simulink model "HEVPlant_Dummy"  (R2018b)
settings: configuration reference "Config_Plant" (kept outside this file)
PreLoadFcn:
  | HEVPlant_Ptbs_V1_BusInfo
model workspace (MAT data in the model file):
  DiffRatio = 3.421
  EV_current = 200
  EV_motion = [20 4 0.8]
  EV_sf = 2000
  EngDriveRatio = 0.813008130081
  Fs = 0
  Fv = 0.0025
  Jcomp = 0.0227
  Jengine = 0.22
  Ki = 251.3274
  Kisa = 346.6583
  Kp_d = 0.47149
  Kp_q = 0.52125
  Ksa = 85.4316
  Ksf = 1996.2651
  Ld = 0.0003752
  Ldq = [0.0003752 0.0004148]
  Lq = 0.0004148
  Mechanical = [0.0227 0.0025 0]
  MotGbRatio = 1
  P = 4
  PolePairs = 4
  RWheel = 0.3
  Rs = 0.2
  T_max = 120
  T_mtpa = [0 13.3131834767 26.6278836885 39.9456159322 53.2678926341 66.5962219318 79.9321062746 93.277041051 106.632513247 120.000000141]
  b_axle = Simulink.Parameter
  b_axle.Value = 10
  b_axle.DataType = 'auto'
  b_axle.Dimensions = [1 1]
  b_driveshaft = Simulink.Parameter
  b_driveshaft.Value = 10
  b_driveshaft.DataType = 'auto'
  b_driveshaft.Dimensions = [1 1]
  ba = 3.4029
  id_mtpa = [0 -0.114523352646 -0.457989076459 -1.03008464374 -1.83029075221 -2.85788367342 -4.11193850568 -5.59133329791 -7.29475400168 -9.22070020138]
  idq0 = [0 0]
  idq_limits = [-9.220699542 166.993501392 167.247872355]
  iq_mtpa = [0 18.5827440345 37.1633719111 55.7397734896 74.3098506185 92.871523015 111.422734008 129.961456105 148.485696337 166.993501356]
  k_axle = Simulink.Parameter
  k_axle.Value = 5000
  k_axle.DataType = 'auto'
  k_axle.Dimensions = [1 1]
  k_driveshaft = Simulink.Parameter
  k_driveshaft.Value = 1000
  k_driveshaft.DataType = 'auto'
  k_driveshaft.Dimensions = [1 1]
  lambda_pm = 0.1194
  mechanical = [0.0227 0.0025 0]
  mot.max_trq = 307
  mot.max_pwr = 124
  mot.spd = [0 500 1000 1500 2000 2500 3000 3500 3857.04487493 4000 4500 5000 5500 6000 6500 7000 7500 8000 8500 9000 9500 10000 10500 11000 11500 12000 12500]
  mot.trq = [307 307 307 307 307 307 307 307 307 296.028194151 263.136172579 236.822555321 215.29323211 197.352129434 182.171196401 169.158968086 157.881703547 148.014097075 139.307385483 131.568086289 124.643450169 118.41127766 112.772645391 107.646616055 102.9663284 98.676064717 94.7290221283]
  mot.trq_cp = [296.028194151 263.136172579 236.822555321 215.29323211 197.352129434 182.171196401 169.158968086 157.881703547 148.014097075 139.307385483 131.568086289 124.643450169 118.41127766 112.772645391 107.646616055 102.9663284 98.676064717 94.7290221283]
  mot.J = 0.02
  mot.damp = 0.0001
  mot.Tc = 0.0267
  mot.map.spdindex = [0 1000 2000 3000 3857 4000 5000 6000 7000 8000 9000 10000 11000 12000 12584]
  mot.map.trqindex = [10 25 50 75 100 125 150 175 200 225 250 275 300 307]
  mot.map.eff = [84  90  90  90  90  90  90  90  90  90  90  90  90  90  90; 84  90  93  95  95  95  96  95  95  95  95  93  93  93  93; 84  90  93  95  95  95  96  95  96  95  95  95  95  93  93; 84  90  93  95  95  95  96  96  96  95  95  95  95  93  93; 84  90  93  95  95  95  96  96  96  95  95  93  93  93  90; 84  88  90  93  93  95  95  96  95  95  95  93  93  93  90; 84  88  90  90  90  93  95  95  95  93  93  93  93  93  90; 84  88  90  90  90  90  93  93  93  93  93  93  93  93  90; 84  84  88  90  90  90  93  93  93  93  93  93  93  93  90; 84  84  88  90  90  90  90  93  93  93  93  93  93  93  90; 84  84  84  90  90  90  90  93  93  93  93  93  93  93  90; 84  84  84  88  90  90  90  93  93  93  93  93  93  93  90; 84  84  84  88  88  88  90  93  93  93  93  93  93  93  90; 84  84  84  88  88  88  90  93  93  93  93  93  93  93  90]
  mot.m = 30
  mot.Cp = 200
  omega_init = 0
  theta_init = 0
  wc_shaft = Simulink.Parameter
  wc_shaft.Value = 0.1
  wc_shaft.DataType = 'auto'
  wc_shaft.Dimensions = [1 1]
libraries: simulink x1
settings Model: Creator=IAEC Nishito  LastModifiedBy=E00026
settings ConfigSetRef: SourceLocation=Base Workspace

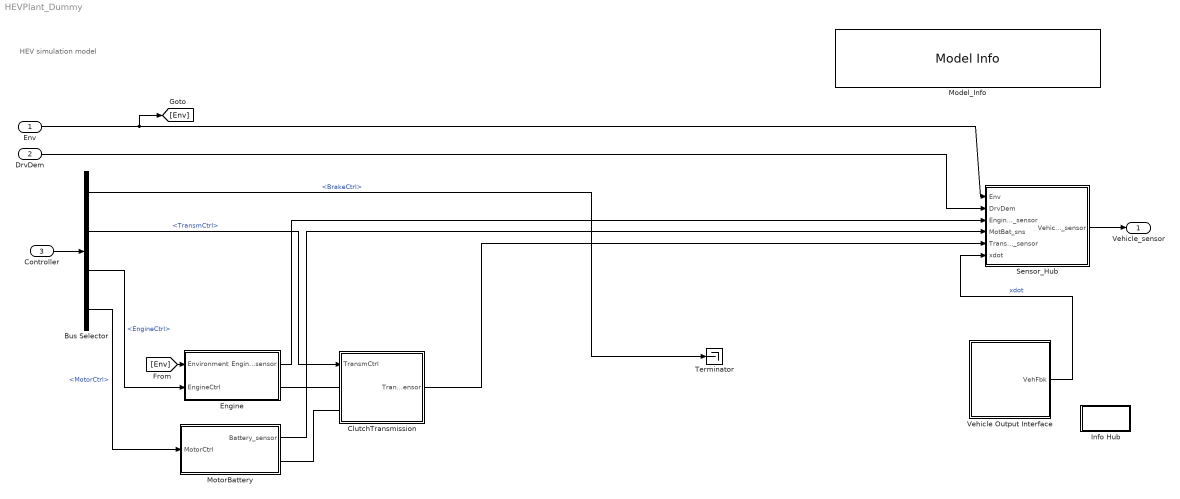
== system HEVPlant_Dummy ==
  note: HEV simulation model
  Env : Inport  OutDataTypeStr=Bus: Environment_Bus
  DrvDem : Inport  Port=2  OutDataTypeStr=Bus: Driver_demand_Bus
  Controller : Inport  Port=3  OutDataTypeStr=Bus: Ctrl_intg_Bus
      settings: AttributesFormatString=%<OutDataTypeStr>
  Bus Selector : BusSelector  OutputSignals=BrakeCtrl,TransmCtrl,EngineCtrl,MotorCtrl
  ClutchTransmission : Subsystem
  Engine : Subsystem
  Info Hub : Subsystem
  Model_Info : simulink/Model-Wide Utilities/Model Info  Frame=on  DisplayStringWithTags=|  HorizontalTextAlignment=Left  LeftAlignmentValue=0.02
      | Version  %<ModelVersion>
      | LastModifided by %<LastModifiedBy>  Date %<LastModificationDate>
      | Description  %<Description>
  MotorBattery : Subsystem
  Sensor_Hub : Subsystem
  Terminator : Terminator
  Vehicle Output Interface : Subsystem
  Vehicle_sensor : Outport  OutDataTypeStr=Bus: Vehicle_sensor_Bus
      settings: AttributesFormatString=%<OutDataTypeStr>
  wires:
  Controller/1 -> Bus Selector/1
  Env/1 -> [Env], Sensor_Hub/1(Env)
  DrvDem/1 -> Sensor_Hub/2(DrvDem)
  Bus Selector/1 -> Terminator/1  "<BrakeCtrl>"
  Bus Selector/4 -> MotorBattery/1(MotorCtrl)  "<MotorCtrl>"
  Bus Selector/2 -> ClutchTransmission/1(TransmCtrl)  "<TransmCtrl>"
  Bus Selector/3 -> Engine/2(EngineCtrl)  "<EngineCtrl>"
  Vehicle Output Interface/1(VehFbk) -> Sensor_Hub/6(xdot)  "xdot"
  MotorBattery/1(Battery_sensor) -> Sensor_Hub/4(MotBat_sns)
  Sensor_Hub/1(Vehicle_sensor) -> Vehicle_sensor/1
  ClutchTransmission/1(Transm_sensor) -> Sensor_Hub/5(Transm_sensor)
  Engine/1(Engine_sensor) -> Sensor_Hub/3(Engine_sensor)
  [Env] -> Engine/1(Environment)
  connections:
  Engine/RConn1 -- ClutchTransmission/LConn1
  MotorBattery/RConn1 -- ClutchTransmission/LConn2

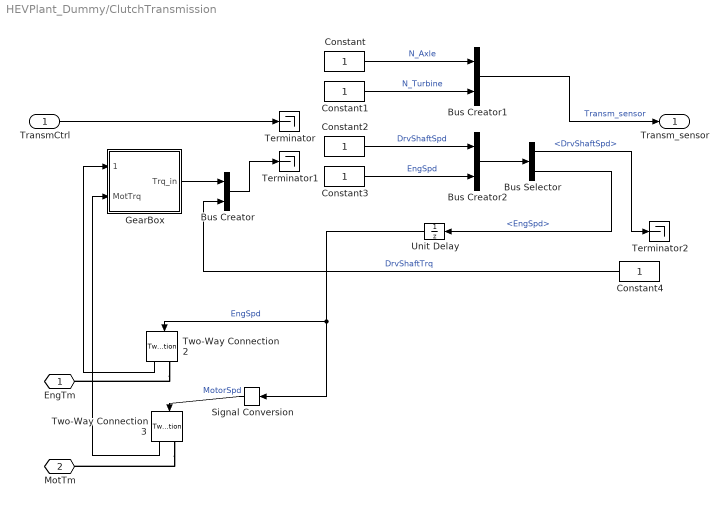
== system HEVPlant_Dummy/ClutchTransmission ==
  TransmCtrl : Inport
  Bus Creator : BusCreator  Inputs=2
  Bus Creator1 : BusCreator  Inputs=2
  Bus Creator2 : BusCreator  Inputs=2
  Bus Selector : BusSelector  OutputSignals=DrvShaftSpd,EngSpd
  Constant{,1..4} (5 alike) : Constant
  GearBox : Subsystem
  Signal Conversion : SignalConversion  OverrideOpt=off
  Terminator : Terminator
  Terminator1 : Terminator
  Terminator2 : Terminator
  Two-Way Connection2 : TwoWayConnection
  Two-Way Connection3 : TwoWayConnection
  Unit Delay : UnitDelay  SampleTime=-1
  EngTm : PMIOPort  Side=Left
  MotTm : PMIOPort  Port=2  Side=Left
  Transm_sensor : Outport
  wires:
  Two-Way Connection3/1 -> GearBox/2(MotTrq)
  Two-Way Connection2/1 -> GearBox/1(EngineTrq)
  Signal Conversion/1 -> Two-Way Connection3/1  "MotorSpd"
  TransmCtrl/1 -> Terminator/1
  GearBox/1(Trq_in) -> Bus Creator/1
  Constant4/1 -> Bus Creator/2  "DrvShaftTrq"
  Bus Creator2/1 -> Bus Selector/1
  Bus Selector/1 -> Terminator2/1  "<DrvShaftSpd>"
  Bus Selector/2 -> Unit Delay/1  "<EngSpd>"
  Bus Creator/1 -> Terminator1/1
  Unit Delay/1 -> Two-Way Connection2/1, Signal Conversion/1  "EngSpd"
  Constant1/1 -> Bus Creator1/2  "N_Turbine"
  Constant/1 -> Bus Creator1/1  "N_Axle"
  Constant2/1 -> Bus Creator2/1  "DrvShaftSpd"
  Constant3/1 -> Bus Creator2/2  "EngSpd"
  Bus Creator1/1 -> Transm_sensor/1  "Transm_sensor"
  connections:
  Two-Way Connection2/RConn1 -- EngTm/RConn1
  Two-Way Connection3/RConn1 -- MotTm/RConn1

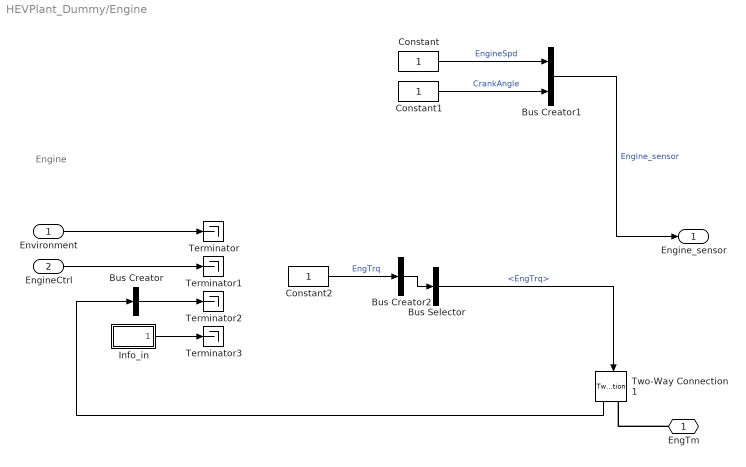
== system HEVPlant_Dummy/Engine ==
  note: Engine
  Environment : Inport
  EngineCtrl : Inport  Port=2
  Bus Creator : BusCreator  Inputs=1
  Bus Creator1 : BusCreator  Inputs=2
  Bus Creator2 : BusCreator  Inputs=1
  Bus Selector : BusSelector  OutputSignals=EngTrq
  Constant : Constant
  Constant1 : Constant
  Constant2 : Constant
  Info_in : Subsystem
  Terminator{,1..3} (4 alike) : Terminator
  Two-Way Connection1 : TwoWayConnection
  EngTm : PMIOPort  Side=Right
  Engine_sensor : Outport
  wires:
  Two-Way Connection1/1 -> Bus Creator/1
  Bus Selector/1 -> Two-Way Connection1/1  "<EngTrq>"
  Environment/1 -> Terminator/1
  EngineCtrl/1 -> Terminator1/1
  Bus Creator/1 -> Terminator2/1
  Info_in/1(Info_in) -> Terminator3/1
  Bus Creator2/1 -> Bus Selector/1
  Constant/1 -> Bus Creator1/1  "EngineSpd"
  Constant1/1 -> Bus Creator1/2  "CrankAngle"
  Bus Creator1/1 -> Engine_sensor/1  "Engine_sensor"
  Constant2/1 -> Bus Creator2/1  "EngTrq"
  connections:
  EngTm/RConn1 -- Two-Way Connection1/RConn1

== system HEVPlant_Dummy/Info Hub ==

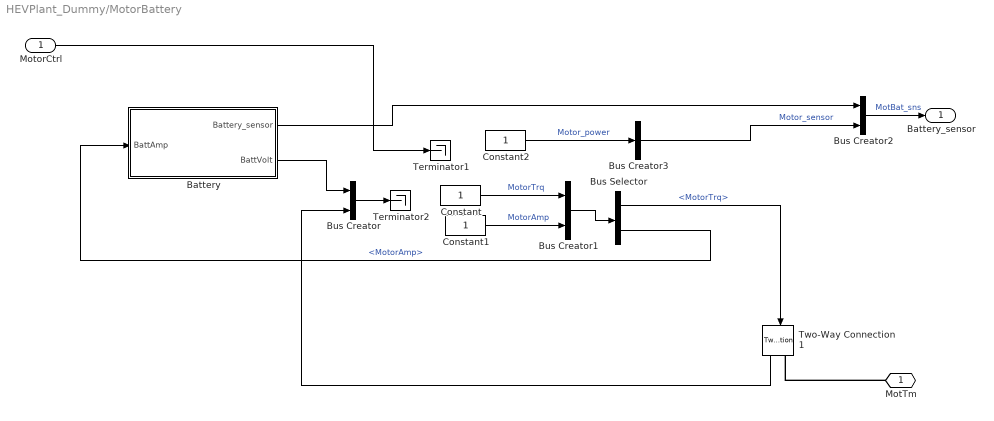
== system HEVPlant_Dummy/MotorBattery ==
  MotorCtrl : Inport
  Battery : Subsystem  TreatAsAtomicUnit=on
  Bus Creator : BusCreator  Inputs=2
  Bus Creator1 : BusCreator  Inputs=2
  Bus Creator2 : BusCreator  Inputs=2
  Bus Creator3 : BusCreator  Inputs=1
  Bus Selector : BusSelector  OutputSignals=MotorTrq,MotorAmp
  Constant : Constant
  Constant1 : Constant
  Constant2 : Constant
  Terminator1 : Terminator
  Terminator2 : Terminator
  Two-Way Connection1 : TwoWayConnection
  MotTm : PMIOPort  Side=Right
  Battery_sensor : Outport
  wires:
  Bus Creator2/1 -> Battery_sensor/1  "MotBat_sns"
  MotorCtrl/1 -> Terminator1/1
  Two-Way Connection1/1 -> Bus Creator/2
  Battery/1(Battery_sensor) -> Bus Creator2/1
  Battery/2(BattVolt) -> Bus Creator/1
  Bus Creator1/1 -> Bus Selector/1
  Bus Selector/1 -> Two-Way Connection1/1  "<MotorTrq>"
  Bus Selector/2 -> Battery/1(BattAmp)  "<MotorAmp>"
  Bus Creator/1 -> Terminator2/1
  Constant1/1 -> Bus Creator1/2  "MotorAmp"
  Constant/1 -> Bus Creator1/1  "MotorTrq"
  Constant2/1 -> Bus Creator3/1  "Motor_power"
  Bus Creator3/1 -> Bus Creator2/2  "Motor_sensor"
  connections:
  MotTm/RConn1 -- Two-Way Connection1/RConn1

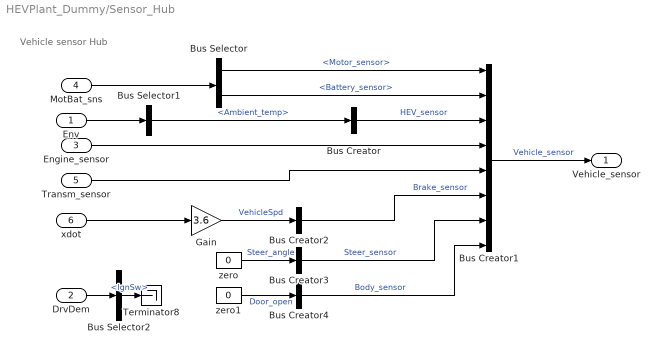
== system HEVPlant_Dummy/Sensor_Hub ==
  note: Vehicle sensor Hub
  Env : Inport
  DrvDem : Inport  Port=2
  Engine_sensor : Inport  Port=3
  MotBat_sns : Inport  Port=4
  Transm_sensor : Inport  Port=5
  xdot : Inport  Port=6
  Bus Creator : BusCreator  Inputs=1  OutDataTypeStr=Bus: HEV_sensor_Bus
      settings: AttributesFormatString=%<OutDataTypeStr>
  Bus Creator1 : BusCreator  Inputs=8  OutDataTypeStr=Bus:Vehicle_sensor_Bus
      settings: AttributesFormatString=%<OutDataTypeStr>
  Bus Creator2 : BusCreator  Inputs=1  OutDataTypeStr=Bus: Brake_sensor_Bus
      settings: AttributesFormatString=%<OutDataTypeStr>
  Bus Creator3 : BusCreator  Inputs=1  OutDataTypeStr=Bus: Steer_sensor_Bus
      settings: AttributesFormatString=%<OutDataTypeStr>
  Bus Creator4 : BusCreator  Inputs=1  OutDataTypeStr=Bus: Body_sensor_Bus
      settings: AttributesFormatString=%<OutDataTypeStr>
  Bus Selector : BusSelector  OutputSignals=Motor_sensor,Battery_sensor
  Bus Selector1 : BusSelector  OutputSignals=Ambient_temp
  Bus Selector2 : BusSelector  OutputSignals=IgnSw
  Gain : Gain  Gain=3.6
  Terminator8 : Terminator
  zero : Constant  Value=0
  zero1 : Constant  Value=0
  Vehicle_sensor : Outport
      settings: AttributesFormatString=%<OutDataTypeStr>
  wires:
  Bus Creator1/1 -> Vehicle_sensor/1  "Vehicle_sensor"
  Engine_sensor/1 -> Bus Creator1/4
  xdot/1 -> Gain/1
  MotBat_sns/1 -> Bus Selector/1
  Bus Selector/1 -> Bus Creator1/1  "<Motor_sensor>"
  Bus Selector/2 -> Bus Creator1/2  "<Battery_sensor>"
  Bus Creator/1 -> Bus Creator1/3  "HEV_sensor"
  Transm_sensor/1 -> Bus Creator1/5
  Gain/1 -> Bus Creator2/1  "VehicleSpd"
  Bus Creator2/1 -> Bus Creator1/6  "Brake_sensor"
  zero/1 -> Bus Creator3/1  "Steer_angle"
  zero1/1 -> Bus Creator4/1  "Door_open"
  Bus Creator3/1 -> Bus Creator1/7  "Steer_sensor"
  Bus Creator4/1 -> Bus Creator1/8  "Body_sensor"
  DrvDem/1 -> Bus Selector2/1
  Env/1 -> Bus Selector1/1
  Bus Selector1/1 -> Bus Creator/1  "<Ambient_temp>"
  Bus Selector2/1 -> Terminator8/1  "<IgnSw>"

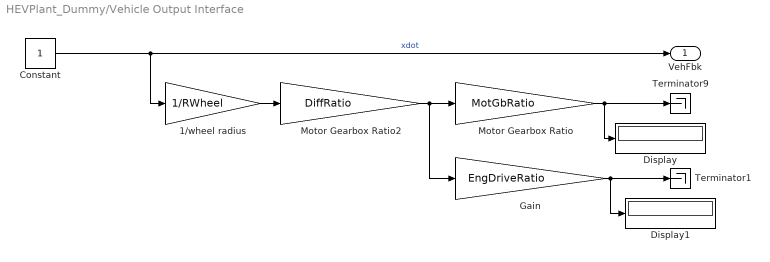
== system HEVPlant_Dummy/Vehicle Output Interface ==
  1/wheel radius : Gain  Gain=1/RWheel
  Constant : Constant
  Display : Display
  Display1 : Display
  Gain : Gain  Gain=EngDriveRatio
  Motor Gearbox Ratio : Gain  Gain=MotGbRatio
  Motor Gearbox Ratio2 : Gain  Gain=DiffRatio
  Terminator1 : Terminator
  Terminator9 : Terminator
  VehFbk : Outport
  wires:
  Gain/1 -> Display1/1, Terminator1/1
  Motor Gearbox Ratio/1 -> Display/1, Terminator9/1
  Motor Gearbox Ratio2/1 -> Gain/1, Motor Gearbox Ratio/1
  1/wheel radius/1 -> Motor Gearbox Ratio2/1
  Constant/1 -> VehFbk/1, 1/wheel radius/1  "xdot"

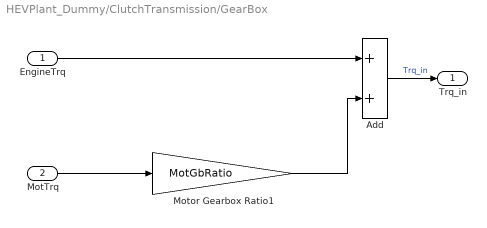
== system HEVPlant_Dummy/ClutchTransmission/GearBox ==
  EngineTrq : Inport
  MotTrq : Inport  Port=2
  Add : Sum
  Motor Gearbox Ratio1 : Gain  Gain=MotGbRatio
  Trq_in : Outport
  wires:
  Add/1 -> Trq_in/1  "Trq_in"
  MotTrq/1 -> Motor Gearbox Ratio1/1
  Motor Gearbox Ratio1/1 -> Add/2
  EngineTrq/1 -> Add/1

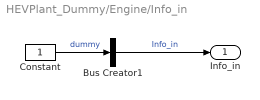
== system HEVPlant_Dummy/Engine/Info_in ==
  Bus Creator1 : BusCreator  Inputs=1
  Constant : Constant
  Info_in : Outport
  wires:
  Constant/1 -> Bus Creator1/1  "dummy"
  Bus Creator1/1 -> Info_in/1  "Info_in"

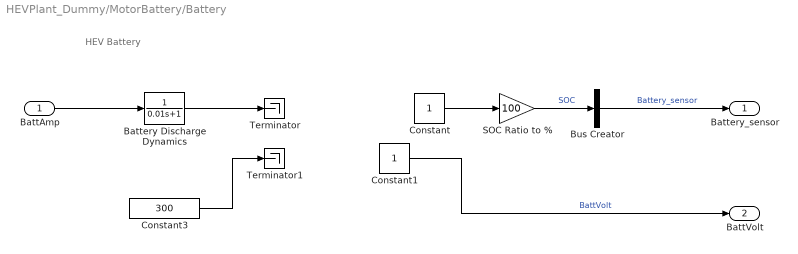
== system HEVPlant_Dummy/MotorBattery/Battery ==
  note: HEV Battery
  BattAmp : Inport
  Battery Discharge Dynamics : TransferFcn  Denominator=[0.01 1]
  Bus Creator : BusCreator  Inputs=1  OutDataTypeStr=Bus: Battery_sensor_Bus
      settings: AttributesFormatString=%<OutDataTypeStr>
  Constant : Constant
  Constant1 : Constant
  Constant3 : Constant  Value=300
  SOC Ratio to % : Gain  Gain=100
  Terminator : Terminator
  Terminator1 : Terminator
  Battery_sensor : Outport
  BattVolt : Outport  Port=2
  wires:
  SOC Ratio to %/1 -> Bus Creator/1  "SOC"
  Constant/1 -> SOC Ratio to %/1
  Constant3/1 -> Terminator1/1
  Battery Discharge Dynamics/1 -> Terminator/1
  Bus Creator/1 -> Battery_sensor/1  "Battery_sensor"
  Constant1/1 -> BattVolt/1  "BattVolt"
  BattAmp/1 -> Battery Discharge Dynamics/1
